simulink model "rover_finalEx"  (R2020b)
settings: Solver=FixedStepAuto  StartTime=0.0  StopTime=inf  FixedStep=TS  RelTol=1e-3  EnableMultiTasking=on
PostLoadFcn:
  | paramsBasicKinematics
  | load('motorResponse.mat')
model workspace (MAT data in the model file):
  TS = 0.01
undefined symbols (not defined in the file): L, PWMcmdMono_L, PWMcmdMono_R, r, speedMono_L, speedMono_R
libraries: arduinowifilib x5, arduinomotorcarrierlib x3, simulink_extras x3, pid_lib x2
settings Model: SILPILModeSetting=veronly  ExtModeTrigDuration=2  Creator=jmodiset  LastModifiedBy=giorg
settings DataIOCC: ReturnWorkspaceOutputs=off
settings OptimizationCC: PassReuseOutputArgsThreshold=0  MaxStackSize=64
settings DebuggingCC: UnderspecifiedInitializationDetection=Classic  MergeDetectMultiDrivingBlocksExec=none  ParameterTunabilityLossMsg=error  PregeneratedLibrarySubsystemCodeDiagnostic=none  ArithmeticOperatorsInVariantConditions=warning
settings HardwareCC: ProdBitPerPointer=32  ProdBitPerSizeT=32  ProdBitPerPtrDiffT=32  ProdLargestAtomicInteger=Long  ProdLargestAtomicFloat=Double  ProdWordSize=32  ProdHWDeviceType=ARM Compatible->ARM Cortex
settings SFSimCC: SimUseLocalCustomCode=off  MATLABDynamicMemAlloc=off  CustomCodeUndefinedFunction=UseInterfaceOnly
settings RTWCC: Description=Embedded Coder  SystemTargetFile=ert.tlc  HardwareBoard=Arduino Nano 33 IoT  TemplateMakefile=ert_default_tmf  RTWUseLocalCustomCode=off  Toolchain=Arduino ARM  BuildConfiguration=Faster Runs
settings CodeAppCC: ForceParamTrailComments=on  OperatorAnnotations=on
settings ERTTargetCC: ERTCustomFileBanners=off  SupportContinuousTime=on  SupportNonInlinedSFcns=on  RemoveResetFunc=off  SupportVariableSizeSignals=on  ModelStepFunctionPrototypeControlCompliant=off  ExtModeStaticAllocSize=8192

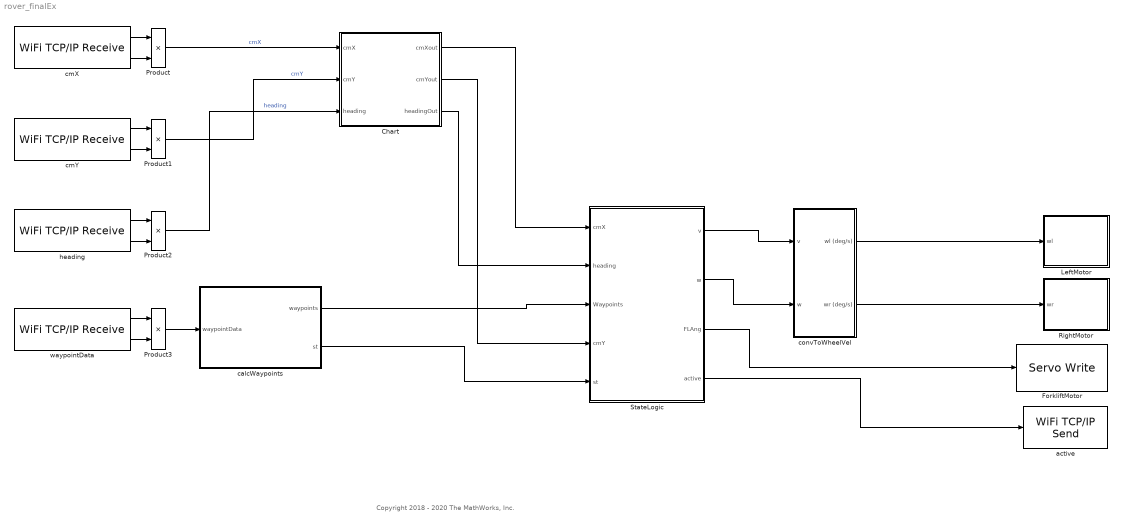
== system rover_finalEx ==
  note: Copyright 2018 - 2020 The MathWorks, Inc.
  Chart : Stateflow chart  TreatAsAtomicUnit=on
  ForkliftMotor : arduinomotorcarrierlib/Servo Write  SlaveAddress=uint8( hex2dec( '66' ) )  blockPlatform=ARDUINO  MotorNumber=3  MotorCarrierPWMFreq=100
      settings: SourceProductBaseCode=ARDUINO
  LeftMotor : Subsystem
      mask Display:
      | color('white');
      | plot([100,100,100,100]*1,[100,100,100,100]*1);
      | plot([100,100,100,100]*0,[100,100,100,100]*0);
      | sppkgroot = strrep(codertarget.arduinobase.internal.getBaseSpPkgRootDir(),'\','/');
      | image(fullfile(sppkgroot,'resources','dcmotor.png'),'center')
  Product{,1..3} (4 alike) : Product
  RightMotor : Subsystem
      mask Display:
      | color('white');
      | plot([100,100,100,100]*1,[100,100,100,100]*1);
      | plot([100,100,100,100]*0,[100,100,100,100]*0);
      | sppkgroot = strrep(codertarget.arduinobase.internal.getBaseSpPkgRootDir(),'\','/');
      | image(fullfile(sppkgroot,'resources','dcmotor.png'),'center')
  StateLogic : Stateflow chart  TreatAsAtomicUnit=on
  active : arduinowifilib/WiFi TCP//IP Send  Mode_=Client  serverport=25005  RemoteAddr_=192.168.137.1  RemoteServerPort_=25005  remoteipoctet1=192  remoteipoctet2=168  remoteipoctet3=137  remoteipoctet4=1  wifiTCPServerIndex=0  wifiTCPClientIndex=0  blockPlatform=ARDUINO  isARMArch=true  SimulateUsing=Code generation
      settings: SourceProductBaseCode=ARDUINO
  calcWaypoints : Stateflow chart  TreatAsAtomicUnit=on
  cmX : arduinowifilib/WiFi TCP//IP Receive  Mode_=Server  serverport=25000  RemoteAddr_=192.168.1.2  RemoteServerPort_=25000  DataType_=double  DataSize_=1  SampleTime_=0.01  remoteipoctet1=192  remoteipoctet2=168  remoteipoctet3=1  remoteipoctet4=2  wifiTCPServerIndex=0  wifiTCPClientIndex=0  blockPlatform=ARDUINO  isARMArch=true  SimulateUsing=Code generation  BlockingMode_=off  BlockTimeout_=0.1
      settings: SourceProductBaseCode=ARDUINO
  cmY : arduinowifilib/WiFi TCP//IP Receive  Mode_=Server  serverport=25001  RemoteAddr_=192.168.1.2  RemoteServerPort_=25000  DataType_=double  DataSize_=1  SampleTime_=0.01  remoteipoctet1=192  remoteipoctet2=168  remoteipoctet3=1  remoteipoctet4=2  wifiTCPServerIndex=1  wifiTCPClientIndex=0  blockPlatform=ARDUINO  isARMArch=true  SimulateUsing=Code generation  BlockingMode_=off  BlockTimeout_=0.1
      settings: SourceProductBaseCode=ARDUINO
  convToWheelVel : Subsystem
  heading : arduinowifilib/WiFi TCP//IP Receive  Mode_=Server  serverport=25002  RemoteAddr_=192.168.1.2  RemoteServerPort_=25000  DataType_=double  DataSize_=1  SampleTime_=0.01  remoteipoctet1=192  remoteipoctet2=168  remoteipoctet3=1  remoteipoctet4=2  wifiTCPServerIndex=2  wifiTCPClientIndex=0  blockPlatform=ARDUINO  isARMArch=true  SimulateUsing=Code generation  BlockingMode_=off  BlockTimeout_=0.1
      settings: SourceProductBaseCode=ARDUINO
  waypointData : arduinowifilib/WiFi TCP//IP Receive  Mode_=Server  serverport=25003  RemoteAddr_=192.168.1.2  RemoteServerPort_=25000  DataType_=double  DataSize_=1  SampleTime_=0.01  remoteipoctet1=192  remoteipoctet2=168  remoteipoctet3=1  remoteipoctet4=2  wifiTCPServerIndex=3  wifiTCPClientIndex=0  blockPlatform=ARDUINO  isARMArch=true  SimulateUsing=Code generation  BlockingMode_=off  BlockTimeout_=0.1
      settings: SourceProductBaseCode=ARDUINO
  wires:
  Product3/1 -> calcWaypoints/1(waypointData)
  StateLogic/4(active) -> active/1
  waypointData/1 -> Product3/1
  convToWheelVel/1(wl (deg/s)) -> LeftMotor/1(wl)
  convToWheelVel/2(wr (deg/s)) -> RightMotor/1(wr)
  Product2/1 -> Chart/3(heading)  "heading"
  calcWaypoints/1(waypoints) -> StateLogic/3(Waypoints)
  calcWaypoints/2(st) -> StateLogic/5(st)
  Chart/1(cmXout) -> StateLogic/1(cmX)
  Chart/3(headingOut) -> StateLogic/2(heading)
  Chart/2(cmYout) -> StateLogic/4(cmY)
  StateLogic/1(v) -> convToWheelVel/1(v)
  StateLogic/3(FLAng) -> ForkliftMotor/1
  heading/2 -> Product2/2
  heading/1 -> Product2/1
  cmX/1 -> Product/1
  Product1/1 -> Chart/2(cmY)  "cmY"
  cmX/2 -> Product/2
  Product/1 -> Chart/1(cmX)  "cmX"
  StateLogic/2(w) -> convToWheelVel/2(w)
  waypointData/2 -> Product3/2
  cmY/2 -> Product1/2
  cmY/1 -> Product1/1

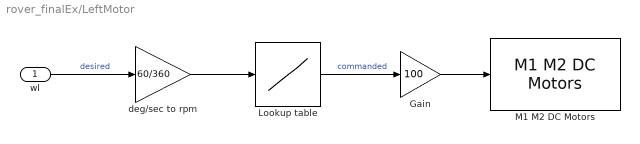
== system rover_finalEx/LeftMotor ==
  wl : Inport
  Gain : Gain  Gain=100
  Lookup table : Lookup_n-D  NumberOfTableDimensions=1  BreakpointsForDimension1=speedMono_L  Table=PWMcmdMono_L  UseLastTableValue=on  InternalRulePriority=Speed  RndMeth=Simplest  InputSameDT=on
  M1 M2 DC Motors : arduinomotorcarrierlib/M1 M2 DC Motors  SlaveAddress=uint8( hex2dec( '66' ) )  blockPlatform=ARDUINO  MotorNumber=M2  MotorCarrierPWMFreq=100
      settings: SourceProductName=Simulink Support Package for Arduino Hardware
  deg/sec to rpm : Gain  Gain=60/360
  wires:
  wl/1 -> deg/sec to rpm/1  "desired"
  Lookup table/1 -> Gain/1  "commanded"
  Gain/1 -> M1 M2 DC Motors/1
  deg/sec to rpm/1 -> Lookup table/1

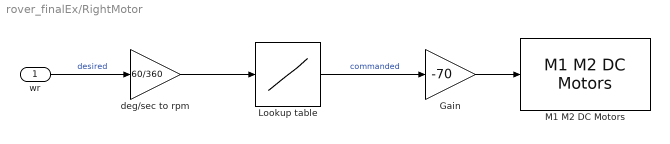
== system rover_finalEx/RightMotor ==
  wr : Inport
  Gain : Gain  Gain=-70
  Lookup table : Lookup_n-D  NumberOfTableDimensions=1  BreakpointsForDimension1=speedMono_R  Table=PWMcmdMono_R  UseLastTableValue=on  InternalRulePriority=Speed  RndMeth=Simplest  InputSameDT=on
  M1 M2 DC Motors : arduinomotorcarrierlib/M1 M2 DC Motors  SlaveAddress=uint8( hex2dec( '66' ) )  blockPlatform=ARDUINO  MotorNumber=M1  MotorCarrierPWMFreq=100
      settings: SourceProductName=Simulink Support Package for Arduino Hardware
  deg/sec to rpm : Gain  Gain=60/360
  wires:
  wr/1 -> deg/sec to rpm/1  "desired"
  Lookup table/1 -> Gain/1  "commanded"
  Gain/1 -> M1 M2 DC Motors/1
  deg/sec to rpm/1 -> Lookup table/1

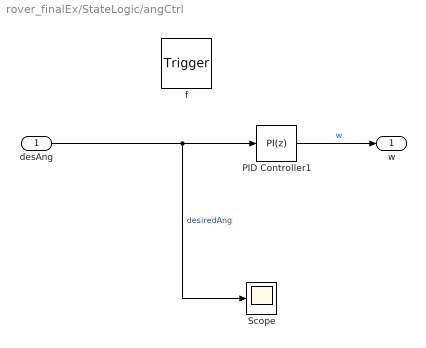
== system rover_finalEx/StateLogic/angCtrl ==
  desAng : Inport  OutDataTypeStr=double  PortDimensions=1
  f : TriggerPort  TriggerType=function-call  VariantControl=(inherit)  PropagateVarSize=Only when enabling  SampleTimeType=periodic  SampleTime=TS
      settings: CopyFcn=Stateflow.SLINSF.SimulinkMan.removeBlockPreDeleteFcn  PreDeleteFcn=Stateflow.SLINSF.SimulinkMan.unsafePredeleteFcn
  PID Controller1 : pid_lib/PID Controller  Controller=PI  Form=Parallel  TimeDomain=Discrete-time  UseExternalTs=off  SampleTime=-1  IntegratorMethod=Forward Euler  FilterMethod=Forward Euler  ControllerParametersSource=internal  P=3  I=1.5  D=0  UseFilter=on  N=100  TunerSelectOption=Transfer Function Based (PID Tuner App)  InitialConditionSource=internal  InitialConditionForIntegrator=0  InitialConditionForFilter=0  DifferentiatorICPrevScaledInput=0  ExternalReset=none  TrackingMode=off  Kt=1  LimitOutput=off  SatLimitsSource=internal  UpperSaturationLimit=inf  LowerSaturationLimit=-inf  LinearizeAsGain=on  AntiWindupMode=none  Kb=1  POutMin=[]  POutMax=[]  IOutMin=[]  IOutMax=[]  DOutMin=[]  DOutMax=[]  NOutMin=[]  NOutMax=[]  SumOutMin=[]  SumOutMax=[]  SaturationOutMin=[]  SaturationOutMax=[]  PParamMin=[]  PParamMax=[]  IParamMin=[]  IParamMax=[]  DParamMin=[]  DParamMax=[]  NParamMin=[]  NParamMax=[]  KbParamMin=[]  KbParamMax=[]  KtParamMin=[]  KtParamMax=[]  KbOutMin=[]  KbOutMax=[]  KtOutMin=[]  KtOutMax=[]  IntegratorOutMin=[]  IntegratorOutMax=[]  FilterOutMin=[]  FilterOutMax=[]  SumI1OutMin=[]  SumI1OutMax=[]  SumI2OutMin=[]  SumI2OutMax=[]  SumI3OutMin=[]  SumI3OutMax=[]  SumI4OutMin=[]  SumI4OutMax=[]  SumDOutMin=[]  SumDOutMax=[]  DifferentiatorOutMin=[]  DifferentiatorOutMax=[]  FilterDiffOutCoefMin=[]  FilterDiffOutCoefMax=[]  ReciprocalOutMin=[]  ReciprocalOutMax=[]  SumDenOutMin=[]  SumDenOutMax=[]  SumNumOutMin=[]  SumNumOutMax=[]  DivideOutMin=[]  DivideOutMax=[]  UdiffTsProdOutMin=[]  UdiffTsProdOutMax=[]  NTsProdOutMin=[]  NTsProdOutMax=[]  UintegralTsProdOutMin=[]  UintegralTsProdOutMax=[]  UngainTsProdOutMin=[]  UngainTsProdOutMax=[]  IntegratorContinuousStateAttributes=''  IntegratorStateMustResolveToSignalObject=off  IntegratorRTWStateStorageClass=Auto  FilterContinuousStateAttributes=''  FilterStateMustResolveToSignalObject=off  FilterRTWStateStorageClass=Auto  ParallelPVariant=InternalParameters  IdealPVariant=Disabled  IVariant=InternalParameters  DVariant=Disabled  IntegratorVariant=Discrete  SatVariant=Disabled  AWVariant=Passthrough  PCopyVariant=Disabled  TRVariant=Disabled  FdbkBlocksVariant=Forward  IdealPFdbkVariant=Disabled  SatFdbkVariant=Disabled  DerivativeFilterVariant=Disabled  NVariant=Disabled  NCopyVariant=Disabled_SignalSpec  FilterICVariant=Disabled  IntegratorICVariant=InternalICs  ExternalResetVariant=Disabled  TRSumVariant=Passthrough  SumFdbkVariant=Disabled  SumVariant=Sum_PI  TsampFilterVariant=InternalTs  TsampNgainVariant=Passthrough  TsampIntegralVariant=Passthrough  ExternalSaturationOutDataTypeStr=Inherit: Same as second input
  Scope : Scope
  w : Outport  VectorParamsAs1DForOutWhenUnconnected=off
  wires:
  desAng/1 -> Scope/1, PID Controller1/1  "desiredAng"
  PID Controller1/1 -> w/1  "w"

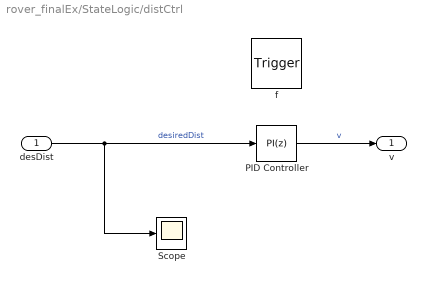
== system rover_finalEx/StateLogic/distCtrl ==
  desDist : Inport  OutDataTypeStr=double  PortDimensions=1
  f : TriggerPort  TriggerType=function-call  VariantControl=(inherit)  PropagateVarSize=Only when enabling  SampleTimeType=periodic  SampleTime=TS
      settings: CopyFcn=Stateflow.SLINSF.SimulinkMan.removeBlockPreDeleteFcn  PreDeleteFcn=Stateflow.SLINSF.SimulinkMan.unsafePredeleteFcn
  PID Controller : pid_lib/PID Controller  Controller=PI  Form=Parallel  TimeDomain=Discrete-time  UseExternalTs=off  SampleTime=-1  IntegratorMethod=Forward Euler  FilterMethod=Forward Euler  ControllerParametersSource=internal  P=2.5  I=0.9  D=0  UseFilter=on  N=100  TunerSelectOption=Transfer Function Based (PID Tuner App)  InitialConditionSource=internal  InitialConditionForIntegrator=0  InitialConditionForFilter=0  DifferentiatorICPrevScaledInput=0  ExternalReset=none  TrackingMode=off  Kt=1  LimitOutput=off  SatLimitsSource=internal  UpperSaturationLimit=inf  LowerSaturationLimit=-inf  LinearizeAsGain=on  AntiWindupMode=none  Kb=1  POutMin=[]  POutMax=[]  IOutMin=[]  IOutMax=[]  DOutMin=[]  DOutMax=[]  NOutMin=[]  NOutMax=[]  SumOutMin=[]  SumOutMax=[]  SaturationOutMin=[]  SaturationOutMax=[]  PParamMin=[]  PParamMax=[]  IParamMin=[]  IParamMax=[]  DParamMin=[]  DParamMax=[]  NParamMin=[]  NParamMax=[]  KbParamMin=[]  KbParamMax=[]  KtParamMin=[]  KtParamMax=[]  KbOutMin=[]  KbOutMax=[]  KtOutMin=[]  KtOutMax=[]  IntegratorOutMin=[]  IntegratorOutMax=[]  FilterOutMin=[]  FilterOutMax=[]  SumI1OutMin=[]  SumI1OutMax=[]  SumI2OutMin=[]  SumI2OutMax=[]  SumI3OutMin=[]  SumI3OutMax=[]  SumI4OutMin=[]  SumI4OutMax=[]  SumDOutMin=[]  SumDOutMax=[]  DifferentiatorOutMin=[]  DifferentiatorOutMax=[]  FilterDiffOutCoefMin=[]  FilterDiffOutCoefMax=[]  ReciprocalOutMin=[]  ReciprocalOutMax=[]  SumDenOutMin=[]  SumDenOutMax=[]  SumNumOutMin=[]  SumNumOutMax=[]  DivideOutMin=[]  DivideOutMax=[]  UdiffTsProdOutMin=[]  UdiffTsProdOutMax=[]  NTsProdOutMin=[]  NTsProdOutMax=[]  UintegralTsProdOutMin=[]  UintegralTsProdOutMax=[]  UngainTsProdOutMin=[]  UngainTsProdOutMax=[]  IntegratorContinuousStateAttributes=''  IntegratorStateMustResolveToSignalObject=off  IntegratorRTWStateStorageClass=Auto  FilterContinuousStateAttributes=''  FilterStateMustResolveToSignalObject=off  FilterRTWStateStorageClass=Auto  ParallelPVariant=InternalParameters  IdealPVariant=Disabled  IVariant=InternalParameters  DVariant=Disabled  IntegratorVariant=Discrete  SatVariant=Disabled  AWVariant=Passthrough  PCopyVariant=Disabled  TRVariant=Disabled  FdbkBlocksVariant=Forward  IdealPFdbkVariant=Disabled  SatFdbkVariant=Disabled  DerivativeFilterVariant=Disabled  NVariant=Disabled  NCopyVariant=Disabled_SignalSpec  FilterICVariant=Disabled  IntegratorICVariant=InternalICs  ExternalResetVariant=Disabled  TRSumVariant=Passthrough  SumFdbkVariant=Disabled  SumVariant=Sum_PI  TsampFilterVariant=InternalTs  TsampNgainVariant=Passthrough  TsampIntegralVariant=Passthrough  ExternalSaturationOutDataTypeStr=Inherit: Same as second input
  Scope : Scope
  v : Outport  VectorParamsAs1DForOutWhenUnconnected=off
  wires:
  desDist/1 -> Scope/1, PID Controller/1  "desiredDist"
  PID Controller/1 -> v/1  "v"

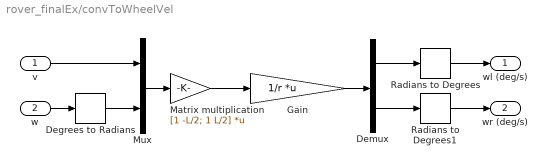
== system rover_finalEx/convToWheelVel ==
  v : Inport
  w : Inport  Port=2
  " Gain" : Gain  Gain=1/r  Multiplication=Matrix(K*u)
  Degrees to Radians : simulink_extras/Transformations/Degrees to Radians
  Demux : Demux  Outputs=2
  Matrix multiplication : Gain  Gain=[1 -L/2; 1 L/2]  Multiplication=Matrix(K*u)
  Mux : Mux  Inputs=2
  Radians to Degrees : simulink_extras/Transformations/Radians to Degrees
  Radians to Degrees1 : simulink_extras/Transformations/Radians to Degrees
  wl (deg/s) : Outport  VectorParamsAs1DForOutWhenUnconnected=off
  wr (deg/s) : Outport  Port=2  VectorParamsAs1DForOutWhenUnconnected=off
  wires:
  " Gain"/1 -> Demux/1
  Matrix multiplication/1 -> " Gain"/1
  v/1 -> Mux/1
  Mux/1 -> Matrix multiplication/1
  Demux/1 -> Radians to Degrees/1
  Demux/2 -> Radians to Degrees1/1
  w/1 -> Degrees to Radians/1
  Radians to Degrees/1 -> wl (deg/s)/1
  Radians to Degrees1/1 -> wr (deg/s)/1
  Degrees to Radians/1 -> Mux/2

== stateflow chart rover_finalEx/calcWaypoints ==
  state waitForCalc
    en, du, ex:
    st = 0;
  state send
    en:
    waypoints = way;
    st = 1;
  state calc
    en:
    way(row, col) = waypointData;
    st = 0;
  state modPos
    en:
    col = 0;
    row = row + 1;
    st = 0;
  (default) -> waitForCalc
  waitForCalc -> send [order 2] : [row > 3]
  modPos -> waitForCalc
  calc -> waitForCalc [order 2]
  waitForCalc -> calc [order 1] : [waypointData ~= 0 && (row <= 3)]{col = col+1}
  calc -> modPos [order 1] : [col >= 2]
  data: waypoints output; waypointData input; row local =1; col local =0; way local =[0 0; 0 0; 0 0]; st output

== stateflow chart rover_finalEx/Chart ==
  state modifyHEADING
    en:
    headingOldValue = heading;
  state Send
    en:
    cmXout = cmXOldValue;
    cmYout = cmYOldValue;
    headingOut = headingOldValue;
  state modifyCMX
    en:
    cmXOldValue = cmX;
  state modifyCMY
    en:
    cmYOldValue = cmY;
  (default) -> Send
  modifyHEADING -> Send
  Send -> modifyCMX [order 1] : [cmX ~= 0]
  Send -> modifyHEADING [order 2] : [heading ~= 0]
  modifyCMX -> Send
  modifyCMY -> Send
  Send -> modifyCMY [order 3] : [cmY ~= 0]
  data: cmX input; cmY input; heading input; cmXout output; cmYout output; headingOut output; cmXOldValue local =0; cmYOldValue local =0; headingOldValue local =0

== stateflow chart rover_finalEx/StateLogic ==
  state Pause
    entry:
    v = 0; w= 0; FLAng = 160;
    active = 1;
  state Pause1
    entry:
    v = 0; w = 0; FLAng = 160;
    active = 1;
  state MoveForwardAndDrop
    state MoveToNextWayPoint
      en:
      desDist = calcDist(WPIndex)-10;
      v = distCtrl(desDist);
      du, ex:
      desDist = calcDist(WPIndex)-10;
      v = distCtrl(desDist);
      w = 0;
    state DropForklift
      en, du, ex:
      v = 0;
      w = 0;
      FLAng = FLAng-1;
    (default) -> MoveForwardAndDrop.MoveToNextWayPoint
    MoveForwardAndDrop.MoveToNextWayPoint -> MoveForwardAndDrop.DropForklift : [abs(desDist) < 6]{WPIndex = WPIndex+1}
  state Turn
    en:
    desAng = calcAngle(WPIndex);
    w = angCtrl(desAng);
    du:
    desAng = calcAngle(WPIndex);
    v = 0;
    w = angCtrl(desAng);
    ex:
    w = 0;
  state w = angCtrl(desAng) [function]
  state MoveForwardAndPickUp
    state MoveToNextWayPoint
      en:
      desDist = calcDist(WPIndex);
      v = distCtrl(desDist);
      du, ex:
      desDist = calcDist(WPIndex);
      v = distCtrl(desDist);
      w = 0;
    state DropForklift
      en, du, ex:
      v = 0;
      w = 0;
      FLAng = FLAng-1;
    state MoveRemaining
      du, ex:
      desDist = calcDist(WPIndex);
      v = distCtrl(desDist);
      w = 0;
    state LiftForklift1
      en, du, ex:
      v = 0;
      w = 0;
      FLAng = FLAng+1;
    (default) -> MoveForwardAndPickUp.MoveToNextWayPoint
    MoveForwardAndPickUp.MoveToNextWayPoint -> MoveForwardAndPickUp.DropForklift : [abs(desDist) < 20]
    MoveForwardAndPickUp.DropForklift -> MoveRemaining : [FLAng < 80]
    MoveRemaining -> LiftForklift1 : [abs(desDist) < 6]{WPIndex = WPIndex+1}
  state v = distCtrl(desDist) [function]
  state Stop
    en:
    v = 0;
    w = 0;
    active = 0;
  MoveForwardAndDrop.DropForklift -> (junction 182) : [FLAng < 80]
  LiftForklift1 -> (junction 182) : [FLAng > 160]
  (default) -> Pause
  Pause -> Pause1 : [st == 1 && cmX ~= 0 && cmY ~= 0]
  Pause1 -> Turn : after(1,sec)
  Turn -> (junction 198) : [abs(desAng) < 8]
  (junction 198) -> MoveForwardAndDrop [order 2] : [WPIndex == 2]
  (junction 198) -> MoveForwardAndPickUp [order 1] : [WPIndex == 1]
  (junction 182) -> Turn [order 2]
  (junction 182) -> Stop [order 1] : [WPIndex == size(Waypoints,1)]
  data: desAngle function_output; Index function_input; desDistance function_output; Index function_input; desAng function_input double size=1; w function_output; desDist function_input double size=1; v function_output; cmX input; heading input; v output double size=1; w output double size=1; desDist local; desAng local; Waypoints input; WPIndex local =1; FLAng output; cmY input; st input; active output
  function desAngle  = calcAngle(Index):
    | function desAngle  = calcAngle(Index)
    | 
    | toReachX = Waypoints(Index+1,1);
    | toReachY = Waypoints(Index+1,2);
    | x = cmX;
    | y = cmY;
    | distX = toReachX - x;
    | distY = toReachY - y;
    | if distX > 0 && distY >= 0
    |     quadrant = 1;
    | elseif distX <= 0 && distY > 0
    |     quadrant = 2;
    | elseif distX < 0 && distY <= 0
    |     quadrant = 3;
    | elseif distX >= 0 && distY < 0
    |     quadrant = 4;
    | else
    |     quadrant = 0;
    | end
    | desAngle = atand((toReachY-y)/(toReachX-x));
    | switch quadrant
    |     case 1
    |         
    |     case 2
    |         desAngle = 180-abs(desAngle);
    |     case 3
    |         desAngle = 180+desAngle;
    |     case 4
    |         desAngle = 360+desAngle;
    |     otherwise 
    |         desAngle = 0;
    | end
    | if desAngle > 360 
    |     desAngle = desAngle - 360;
    | end
    | 
    | desAngle = desAngle - 180;      %conversion needed to avoid the offset of 
    |                                 %the value compared to heading
    | desAngle = desAngle + heading;  %the angle to face the target
    | 
    |  if(desAngle > 180)             %conversions to avoid spinning too much
    |    desAngle = desAngle - 360;
    |  elseif(desAngle < -180)
    |      desAngle = desAngle + 360;
    |  end
    | end
  function desDistance = calcDist(Index):
    | function desDistance = calcDist(Index)
    | 
    | toReachX = Waypoints(Index+1,1);
    | toReachY = Waypoints(Index+1,2);
    | x = cmX;
    | y = cmY;
    | distX = toReachX - x;
    | distY = toReachY - y;
    | desDistance = sqrt(distX^2+distY^2);
    | end
